simulink model "Gyro_Reading"  (R2022b)
settings: Solver=FixedStepDiscrete  StartTime=0.0  StopTime=inf  RelTol=1e-3  EnableMultiTasking=on
InitFcn:
  | run("InitScript.m");
undefined symbols (not defined in the file or in its folder): A_cal, b_cal, ODR, operatingFrequency
libraries: hdlsllib x12, mbedblockslib x10, simulink x6, aerolibanim x1
settings Model: ExtModeTrigDuration=10  Creator=rutrl  LastModifiedBy=rutrl
settings OptimizationCC: EnhancedBackFolding=on  PassReuseOutputArgsAs=Individual arguments  ZeroExternalMemoryAtStartup=off  ZeroInternalMemoryAtStartup=off  MaxStackSize=64  OptimizeBlockOrder=speed  DifferentSizesBufferReuse=on  OptimizationCustomize=off  EfficientTunableParamExpr=on
settings DebuggingCC: ParameterTunabilityLossMsg=error
settings HardwareCC: ProdBitPerPointer=32  ProdBitPerSizeT=32  ProdBitPerPtrDiffT=32  ProdLargestAtomicInteger=Long  ProdLargestAtomicFloat=Double  ProdWordSize=32  ProdLongLongMode=on  ProdHWDeviceType=ARM Compatible->ARM Cortex  UseEmbeddedCoderFeatures=off
settings SFSimCC: MATLABDynamicMemAlloc=off
settings RTWCC: Description=Embedded Coder  SystemTargetFile=ert.tlc  HardwareBoard=STM32 Nucleo L476RG  TLCOptions=-aInlineSetEventsForThisBaseRateFcn=TLC_FALSE -aSuppressMultiTaskScheduler=TLC_FALSE -aRateBasedStepFcn=1  TemplateMakefile=ert_default_tmf  Toolchain=GNU Tools for ARM Embedded Processors
settings CodeAppCC: ForceParamTrailComments=on  IgnoreCustomStorageClasses=off  OperatorAnnotations=on  SimulinkDataObjDesc=on  SFDataObjDesc=on  InsertBlockDesc=on
settings ERTTargetCC: SupportNonInlinedSFcns=on  ExtModeTransport=3  ExtModeStaticAlloc=on  ExtModeStaticAllocSize=2000  ExtModeMexFile=ext_xcp  ExtModeIntrfLevel=Level2 - Open

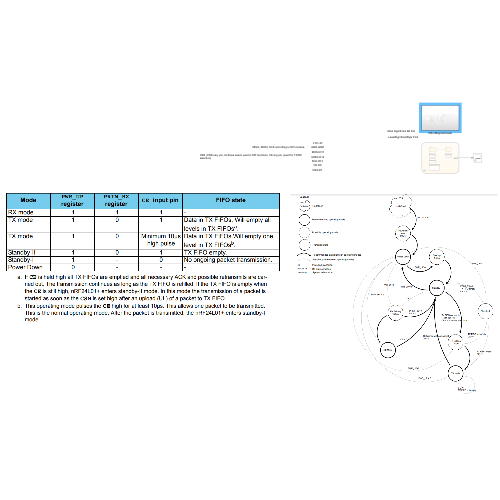
[thumbnail: Simulink's stored preview of the top-level diagram]
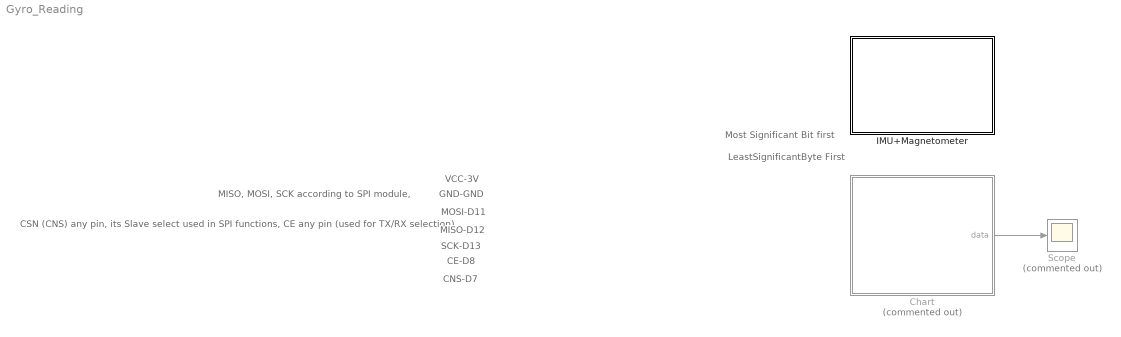
== system Gyro_Reading ==
  note: LeastSignificantByte First
  note: CNS-D7
  note: CSN (CNS) any pin, its Slave select used in SPI functions, CE any pin (used for TX/RX selection)
  note: MISO, MOSI, SCK according to SPI module,
  note: Most Significant Bit first
  note: CE-D8
  note: SCK-D13
  note: MISO-D12
  note: MOSI-D11
  note: GND-GND
  note: VCC-3V
  Chart : Stateflow chart  Commented=on  TreatAsAtomicUnit=on
  IMU+Magnetometer : Subsystem
  Scope : Scope  Commented=on
  wires:
  Chart/1(data) -> Scope/1

== system Gyro_Reading/Chart/? ==
  f : TriggerPort  TriggerType=function-call  VariantControl=(inherit)
      settings: CopyFcn=Stateflow.SLINSF.SimulinkMan.removeBlockPreDeleteFcn  PreDeleteFcn=Stateflow.SLINSF.SimulinkMan.unsafePredeleteFcn

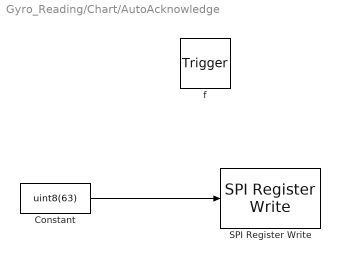
== system Gyro_Reading/Chart/AutoAcknowledge ==
  f : TriggerPort  TriggerType=function-call  VariantControl=(inherit)
      settings: CopyFcn=Stateflow.SLINSF.SimulinkMan.removeBlockPreDeleteFcn  PreDeleteFcn=Stateflow.SLINSF.SimulinkMan.unsafePredeleteFcn
  Constant : Constant  Value=uint8(63)
  SPI Register Write : mbedblockslib/SPI Register Write  SPIModule=0  Mode=Master  BusSpeed=uint32( 1000000 )  Pin=D7  FirstBitToTransfer=Most significant bit (MSB)  ClockMode=0  BlockFunction=Write  RegisterAddress=uint8(hex2dec('01'))  OutputDataType=int8  OutputDataLength=1  UseCustomSSPin=Explicit GPIO calls  ActiveLowSSPin=Active low
      settings: LibrarySourceBlock=stmnucleorootlib/Common/SPI Register Write
  wires:
  Constant/1 -> SPI Register Write/1

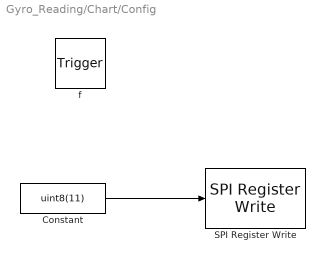
== system Gyro_Reading/Chart/Config ==
  f : TriggerPort  TriggerType=function-call  VariantControl=(inherit)
      settings: CopyFcn=Stateflow.SLINSF.SimulinkMan.removeBlockPreDeleteFcn  PreDeleteFcn=Stateflow.SLINSF.SimulinkMan.unsafePredeleteFcn
  Constant : Constant  Value=uint8(11)
  SPI Register Write : mbedblockslib/SPI Register Write  SPIModule=0  Mode=Master  BusSpeed=uint32( 1000000 )  Pin=D7  FirstBitToTransfer=Most significant bit (MSB)  ClockMode=0  BlockFunction=Write  RegisterAddress=uint8(hex2dec('00'))  OutputDataType=int8  OutputDataLength=1  UseCustomSSPin=Explicit GPIO calls  ActiveLowSSPin=Active low
      settings: LibrarySourceBlock=stmnucleorootlib/Common/SPI Register Write
  wires:
  Constant/1 -> SPI Register Write/1

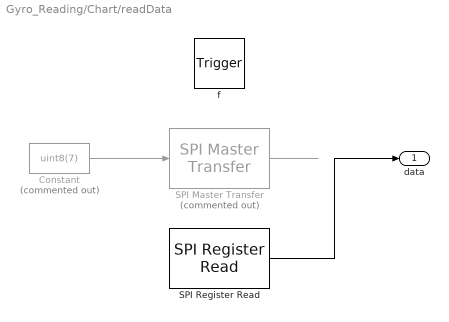
== system Gyro_Reading/Chart/readData ==
  f : TriggerPort  TriggerType=function-call  VariantControl=(inherit)
      settings: CopyFcn=Stateflow.SLINSF.SimulinkMan.removeBlockPreDeleteFcn  PreDeleteFcn=Stateflow.SLINSF.SimulinkMan.unsafePredeleteFcn
  Constant : Constant  Commented=on  Value=uint8(7)
  SPI Master Transfer : mbedblockslib/SPI Master Transfer  Commented=on  SPIModule=0  Mode=Master  BusSpeed=uint32( 1000000 )  Pin=D7  FirstBitToTransfer=Most significant bit (MSB)  ClockMode=0  BlockFunction=Transfer  RegisterAddress=0  OutputDataType=int8  OutputDataLength=1  UseCustomSSPin=Explicit GPIO calls  ActiveLowSSPin=Active low
      settings: LibrarySourceBlock=stmnucleorootlib/Common/SPI Master Transfer
  SPI Register Read : mbedblockslib/SPI Register Read  SPIModule=0  Mode=Master  BusSpeed=uint32( 1000000 )  Pin=D7  FirstBitToTransfer=Most significant bit (MSB)  ClockMode=0  BlockFunction=Read  RegisterAddress=uint8(hex2dec('07'))  OutputDataType=uint8  OutputDataLength=1  SampleTime=-1  UseCustomSSPin=Explicit GPIO calls  ActiveLowSSPin=Active low
      settings: LibrarySourceBlock=stmnucleorootlib/Common/SPI Register Read
  data : Outport
  wires:
  SPI Master Transfer/1 -> ?
  Constant/1 -> SPI Master Transfer/1
  SPI Register Read/1 -> data/1

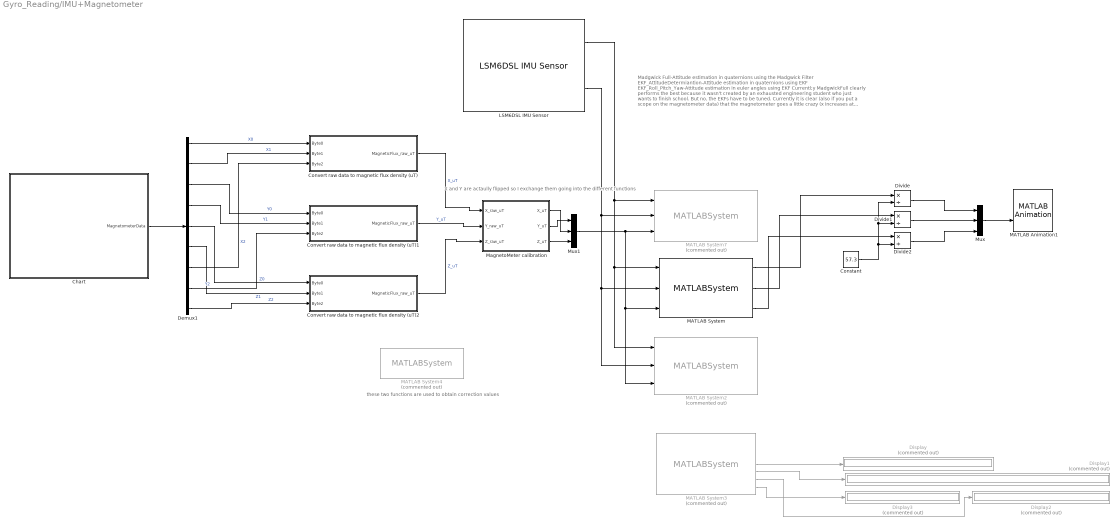
== system Gyro_Reading/IMU+Magnetometer ==
  note: Madgwick Full-Attitude estimation in quaternions using the Madgwick Filter
      | EKF_AttitudeDetermiantion-Attitude estimation in quaternions using EKF
      | EKF_Roll_Pitch_Yaw-Attitude estimation in euler angles using EKF
      |
      | Currentl;y MadgwickFull clearly performs the best because it wasn't created by
      | an exhausted engineering student who just wants to finish school. But no, the
      | EKFs have to be tuned. Currently it is clear (also if you put a scope on the
      | magnetometer data) that the magnetometer goes a little crazy (x increases at higher rate than y (or the other way around) so it mathematically results in change of yaw but then it settles at the appropriate values again once the speed decreases) at higher angular speeds.
      | Hence it is worth the time to try to come up with a function that will estiamte the most appropriate Q and R values based on the angular speed, such that at higher speeds we rely more on the gyroscope (prediction) and at lower speed we rely more on the magnetometer (update)
      |
      | In conclusion, these can be used as prrof of concept for further development.
  note: X and Y are actaully flipped so I exchange them going into the different functions
  note: these two functions are used to obtain correction values
  Chart : Stateflow chart  TreatAsAtomicUnit=on
  Constant : Constant  Value=57.3
  Convert raw data to magnetic flux density (uT) : Subsystem
  Convert raw data to magnetic flux density (uT)1 : Subsystem
  Convert raw data to magnetic flux density (uT)2 : Subsystem
  Demux1 : Demux  Outputs=9
  Display{,1..3} (4 alike) : Display  Commented=on
  Divide : Product  Inputs=*/
  Divide1 : Product  Inputs=*/
  Divide2 : Product  Inputs=*/
  LSM6DSL IMU Sensor : mbedblockslib/LSM6DSL IMU Sensor  I2CModule=0  I2CAddress=0x6A  IsActiveAcceleration=on  IsActiveAngularRate=on  IsActiveTemperature=off  IsActiveStatus=off  IsActiveTimeStamp=off  SampleTime=1/operatingFrequency  QueueSizeFactor=3  AccelerometerRange=+/- 8g  AccelerometerODR=208 Hz  AccelLPF1BW=ODR/4  AccelSelectCompositeFilter=Low pass filter  AccelLPF2BW=ODR/100  AccelHPFBW=ODR/100  GyroscopeRange=1000 dps  GyroscopeODR=208 Hz  EnableGyroHPF=off  GyroHPFBW=0.016 Hz  EnableGyroLPF=on  GyroLPFBWMode=3
      settings: LibrarySourceBlock=stmnucleosensorslib/LSM6DSL IMU Sensor
  MATLAB Animation1 : aerolibanim/MATLAB Animation  Tag=Matlab Animation 6 DOF  Vehicles=1  Geometries='astredwedge.mat'  BoundingBoxCoordinates=[-50,50,-50,50,-50,50]  CameraOffset=[-150,-50,0]  CameraViewAngle=3  SampleTime=-1  FigurePosition=[529,285,1158,525]
  MATLAB System : MATLABSystem  System=EKF_AttitudeDetermination  samplingFrequency=operatingFrequency  gyro_x_corr=gyro_x_corr  gyro_y_corr=gyro_y_corr  gyro_z_corr=gyro_z_corr  SimulateUsing=Code generation
      mask Type: EKF_AttitudeDetermination
      mask Display:
      | disp('EKF_AttitudeDetermination');
      | port_label('input',1,'accelerometer');
      | port_label('input',2,'gyroscope');
      | port_label('input',3,'magnetometer');
      | port_label('output',1,'roll');
      | port_label('output',2,'pitch');
      | port_label('output',3,'yaw');
  MATLAB System2 : MATLABSystem  Commented=on  System=EKF_Roll_Pitch_Yaw  samplingFrequency=operatingFrequency  gyro_x_corr=gyro_x_corr  gyro_y_corr=gyro_y_corr  gyro_z_corr=gyro_z_corr  SimulateUsing=Code generation
      mask Type: EKF_Roll_Pitch_Yaw
      mask Display:
      | disp('EKF_Roll_Pitch_Yaw');
      | port_label('input',1,'accelerometer');
      | port_label('input',2,'gyroscope');
      | port_label('input',3,'magnetometer');
      | port_label('output',1,'roll');
      | port_label('output',2,'pitch');
      | port_label('output',3,'yaw');
  MATLAB System3 : MATLABSystem  Commented=on  System=EKF_Testing  samplingFrequency=operatingFrequency  gyro_x_corr=gyro_x_corr  gyro_y_corr=gyro_y_corr  gyro_z_corr=gyro_z_corr  SimulateUsing=Code generation
      mask Type: EKF_Testing
      mask Display:
      | disp('EKF_Testing');
      | port_label('input',1,'accelerometer');
      | port_label('input',2,'gyroscope');
      | port_label('input',3,'magnetometer');
      | port_label('output',1,'roll');
      | port_label('output',2,'pitch');
      | port_label('output',3,'yaw');
      | port_label('output',4,'q');
      | port_label('output',5,'h');
      | port_label('output',6,'m_prime');
      | port_label('output',7,'a');
  MATLAB System4 : MATLABSystem  Commented=on  System=GyroCorr  operatingFrequency=operatingFrequency  SimulateUsing=Code generation
      mask Type: GyroCorr
      mask Display:
      | disp('GyroCorr');
      | port_label('input',1,'gyroscope');
      | port_label('output',1,'gyro_x');
      | port_label('output',2,'gyro_y');
      | port_label('output',3,'gyro_z');
  MATLAB System7 : MATLABSystem  Commented=on  System=MadgwickFull  samplingFrequency=operatingFrequency  gyro_x_corr=gyro_x_corr  gyro_y_corr=gyro_y_corr  gyro_z_corr=gyro_z_corr  SimulateUsing=Code generation
      mask Type: MadgwickFull
      mask Display:
      | disp('MadgwickFull');
      | port_label('input',1,'accelerometer');
      | port_label('input',2,'gyroscope');
      | port_label('input',3,'magnetometer');
      | port_label('output',1,'roll');
      | port_label('output',2,'pitch');
      | port_label('output',3,'yaw');
  MagnetoMeter calibration : Subsystem
  Mux : Mux  Inputs=3
  Mux1 : Mux  Inputs=3
  wires:
  Demux1/5 -> Convert raw data to magnetic flux density (uT)2/1(Byte0)  "Z0"
  Demux1/9 -> Convert raw data to magnetic flux density (uT)2/3(Byte2)  "Z2"
  Convert raw data to magnetic flux density (uT)2/1(MagneticFlux_raw_uT) -> MagnetoMeter calibration/3(Z_raw_uT)  "Z_uT"
  Demux1/4 -> Convert raw data to magnetic flux density (uT)1/2(Byte1)  "Y1"
  Convert raw data to magnetic flux density (uT)/1(MagneticFlux_raw_uT) -> MagnetoMeter calibration/1(X_raw_uT)  "X_uT"
  Demux1/6 -> Convert raw data to magnetic flux density (uT)2/2(Byte1)  "Z1"
  Demux1/1 -> Convert raw data to magnetic flux density (uT)/1(Byte0)  "X0"
  Demux1/7 -> Convert raw data to magnetic flux density (uT)/3(Byte2)  "X2"
  Convert raw data to magnetic flux density (uT)1/1(MagneticFlux_raw_uT) -> MagnetoMeter calibration/2(Y_raw_uT)  "Y_uT"
  Demux1/8 -> Convert raw data to magnetic flux density (uT)1/3(Byte2)  "Y2"
  Demux1/2 -> Convert raw data to magnetic flux density (uT)/2(Byte1)  "X1"
  Chart/1(MagnetometerData) -> Demux1/1
  Demux1/3 -> Convert raw data to magnetic flux density (uT)1/1(Byte0)  "Y0"
  LSM6DSL IMU Sensor/2 -> MATLAB System7/2, MATLAB System/2, MATLAB System2/2
  LSM6DSL IMU Sensor/1 -> MATLAB System7/1, MATLAB System/1, MATLAB System2/1
  Constant/1 -> Divide/2, Divide1/2, Divide2/2
  Divide1/1 -> Mux/2
  MagnetoMeter calibration/1(X_uT) -> Mux1/2
  MagnetoMeter calibration/2(Y_uT) -> Mux1/1
  MagnetoMeter calibration/3(Z_uT) -> Mux1/3
  Mux/1 -> MATLAB Animation1/2
  Divide/1 -> Mux/1
  Divide2/1 -> Mux/3
  MATLAB System3/4 -> Display/1
  MATLAB System3/5 -> Display1/1
  MATLAB System3/6 -> Display2/1
  MATLAB System3/7 -> Display3/1
  Mux1/1 -> MATLAB System2/3, MATLAB System/3, MATLAB System7/3
  MATLAB System/1 -> Divide/1
  MATLAB System/2 -> Divide1/1
  MATLAB System/3 -> Divide2/1

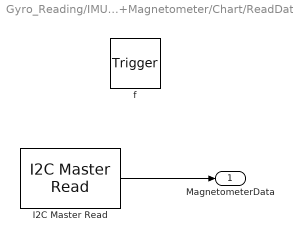
== system Gyro_Reading/IMU+Magnetometer/Chart/ReadData ==
  f : TriggerPort  TriggerType=function-call  VariantControl=(inherit)
      settings: CopyFcn=Stateflow.SLINSF.SimulinkMan.removeBlockPreDeleteFcn  PreDeleteFcn=Stateflow.SLINSF.SimulinkMan.unsafePredeleteFcn
  I2C Master Read : mbedblockslib/I2C Master Read  I2CModule=0  Mode=Master  SlaveAddress=hex2dec('30')  SlaveByteOrder=LittleEndian  Direction=Receiver  RegisterAddressMode=on  RegisterAddress=uint8(hex2dec('00'))  SlaveDataType=uint8  DataLength=9  NoAck=off  RepeatedStart=off  OutputStatus=off  SampleTime=-1
      settings: LibrarySourceBlock=stmnucleorootlib/Common/I2C Master Read
  MagnetometerData : Outport
  wires:
  I2C Master Read/1 -> MagnetometerData/1

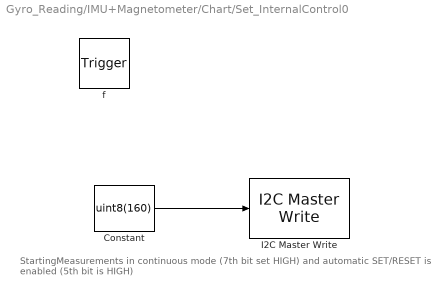
== system Gyro_Reading/IMU+Magnetometer/Chart/Set_InternalControl0 ==
  note: StartingMeasurements in continuous mode (7th bit set HIGH) and automatic SET/RESET is enabled (5th bit is HIGH)
  f : TriggerPort  TriggerType=function-call  VariantControl=(inherit)
      settings: CopyFcn=Stateflow.SLINSF.SimulinkMan.removeBlockPreDeleteFcn  PreDeleteFcn=Stateflow.SLINSF.SimulinkMan.unsafePredeleteFcn
  Constant : Constant  Value=uint8(160)
  I2C Master Write : mbedblockslib/I2C Master Write  I2CModule=0  Mode=Master  SlaveAddress=hex2dec('30')  SlaveByteOrder=BigEndian  Direction=Transmitter  RegisterAddressMode=on  RegisterAddress=uint8(hex2dec('1B'))  SlaveDataType=uint8  DataLength=2  NoAck=off  RepeatedStart=off  OutputStatus=off
      settings: LibrarySourceBlock=stmnucleorootlib/Common/I2C Master Write
  wires:
  Constant/1 -> I2C Master Write/1

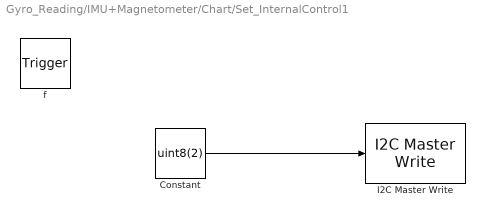
== system Gyro_Reading/IMU+Magnetometer/Chart/Set_InternalControl1 ==
  f : TriggerPort  TriggerType=function-call  VariantControl=(inherit)
      settings: CopyFcn=Stateflow.SLINSF.SimulinkMan.removeBlockPreDeleteFcn  PreDeleteFcn=Stateflow.SLINSF.SimulinkMan.unsafePredeleteFcn
  Constant : Constant  Value=uint8(2)
  I2C Master Write : mbedblockslib/I2C Master Write  I2CModule=0  Mode=Master  SlaveAddress=hex2dec('30')  SlaveByteOrder=BigEndian  Direction=Transmitter  RegisterAddressMode=on  RegisterAddress=uint8(hex2dec('1C'))  SlaveDataType=uint8  DataLength=2  NoAck=off  RepeatedStart=off  OutputStatus=off
      settings: LibrarySourceBlock=stmnucleorootlib/Common/I2C Master Write
  wires:
  Constant/1 -> I2C Master Write/1

== system Gyro_Reading/IMU+Magnetometer/Chart/Set_InternalControl2 ==
  note: Just setting continuous mode to 1
  f : TriggerPort  TriggerType=function-call  VariantControl=(inherit)
      settings: CopyFcn=Stateflow.SLINSF.SimulinkMan.removeBlockPreDeleteFcn  PreDeleteFcn=Stateflow.SLINSF.SimulinkMan.unsafePredeleteFcn
  Constant : Constant  Value=uint8(16)
  I2C Master Write : mbedblockslib/I2C Master Write  I2CModule=0  Mode=Master  SlaveAddress=hex2dec('30')  SlaveByteOrder=BigEndian  Direction=Transmitter  RegisterAddressMode=on  RegisterAddress=uint8(hex2dec('1D'))  SlaveDataType=uint8  DataLength=2  NoAck=off  RepeatedStart=off  OutputStatus=off
      settings: LibrarySourceBlock=stmnucleorootlib/Common/I2C Master Write
  wires:
  Constant/1 -> I2C Master Write/1

== system Gyro_Reading/IMU+Magnetometer/Chart/Set_ODR ==
  note: Just put desired frequency into bracket. BW is set to 10 in internal control 1
  f : TriggerPort  TriggerType=function-call  VariantControl=(inherit)
      settings: CopyFcn=Stateflow.SLINSF.SimulinkMan.removeBlockPreDeleteFcn  PreDeleteFcn=Stateflow.SLINSF.SimulinkMan.unsafePredeleteFcn
  Constant : Constant  Value=uint8(200)
  I2C Master Write : mbedblockslib/I2C Master Write  I2CModule=0  Mode=Master  SlaveAddress=hex2dec('30')  SlaveByteOrder=BigEndian  Direction=Transmitter  RegisterAddressMode=on  RegisterAddress=uint8(hex2dec('1A'))  SlaveDataType=uint8  DataLength=2  NoAck=off  RepeatedStart=off  OutputStatus=off
      settings: LibrarySourceBlock=stmnucleorootlib/Common/I2C Master Write
  wires:
  Constant/1 -> I2C Master Write/1

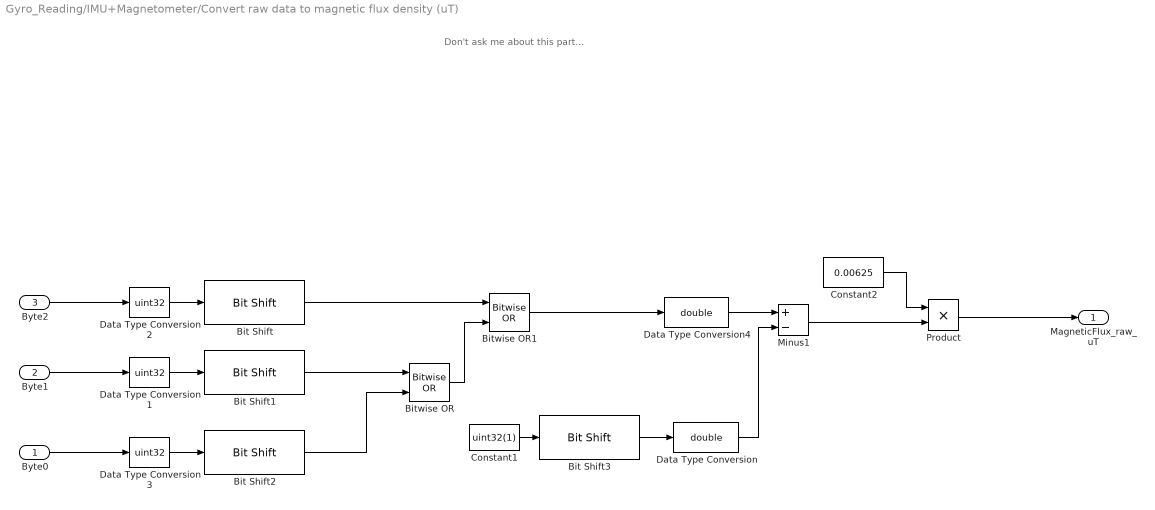
== system Gyro_Reading/IMU+Magnetometer/Convert raw data to magnetic flux density (uT) ==
  note: Don't ask me about this part...
  Byte0 : Inport
  Byte1 : Inport  Port=2
  Byte2 : Inport  Port=3
  Bit Shift : hdlsllib/Logic and Bit Operations/Bit Shift  mode=Shift Right Logical  N=4
  Bit Shift1 : hdlsllib/Logic and Bit Operations/Bit Shift  mode=Shift Left Logical  N=4
  Bit Shift2 : hdlsllib/Logic and Bit Operations/Bit Shift  mode=Shift Left Logical  N=12
  Bit Shift3 : hdlsllib/Logic and Bit Operations/Bit Shift  mode=Shift Left Logical  N=19
  Bitwise OR : simulink/Logic and Bit Operations/Bitwise Operator  logicop=OR  UseBitMask=off  NumInputPorts=2  BitMask=bin2dec('11011001')  BitMaskRealWorld=Stored Integer
      settings: LibrarySourceBlock=|
      | simulink/Quick Insert/Logic and Bit
      | Operations/Bitwise OR
  Bitwise OR1 : simulink/Logic and Bit Operations/Bitwise Operator  logicop=OR  UseBitMask=off  NumInputPorts=2  BitMask=bin2dec('11011001')  BitMaskRealWorld=Stored Integer
      settings: LibrarySourceBlock=|
      | simulink/Quick Insert/Logic and Bit
      | Operations/Bitwise OR
  Constant1 : Constant  Value=uint32(1)
  Constant2 : Constant  Value=0.00625
  Data Type Conversion : DataTypeConversion  OutDataTypeStr=double  SaturateOnIntegerOverflow=off  RndMeth=Floor
  Data Type Conversion1 : DataTypeConversion  OutDataTypeStr=uint32  SaturateOnIntegerOverflow=off  RndMeth=Floor
  Data Type Conversion2 : DataTypeConversion  OutDataTypeStr=uint32  SaturateOnIntegerOverflow=off  RndMeth=Floor
  Data Type Conversion3 : DataTypeConversion  OutDataTypeStr=uint32  SaturateOnIntegerOverflow=off  RndMeth=Floor
  Data Type Conversion4 : DataTypeConversion  OutDataTypeStr=double  SaturateOnIntegerOverflow=off  RndMeth=Floor
  Minus1 : Sum  Inputs=+-
  Product : Product
  MagneticFlux_raw_uT : Outport
  wires:
  Bit Shift/1 -> Bitwise OR1/1
  Bit Shift2/1 -> Bitwise OR/2
  Data Type Conversion3/1 -> Bit Shift2/1
  Byte0/1 -> Data Type Conversion3/1
  Bit Shift1/1 -> Bitwise OR/1
  Bitwise OR1/1 -> Data Type Conversion4/1
  Constant1/1 -> Bit Shift3/1
  Bitwise OR/1 -> Bitwise OR1/2
  Data Type Conversion2/1 -> Bit Shift/1
  Minus1/1 -> Product/2
  Byte1/1 -> Data Type Conversion1/1
  Bit Shift3/1 -> Data Type Conversion/1
  Data Type Conversion1/1 -> Bit Shift1/1
  Product/1 -> MagneticFlux_raw_uT/1
  Constant2/1 -> Product/1
  Byte2/1 -> Data Type Conversion2/1
  Data Type Conversion/1 -> Minus1/2
  Data Type Conversion4/1 -> Minus1/1

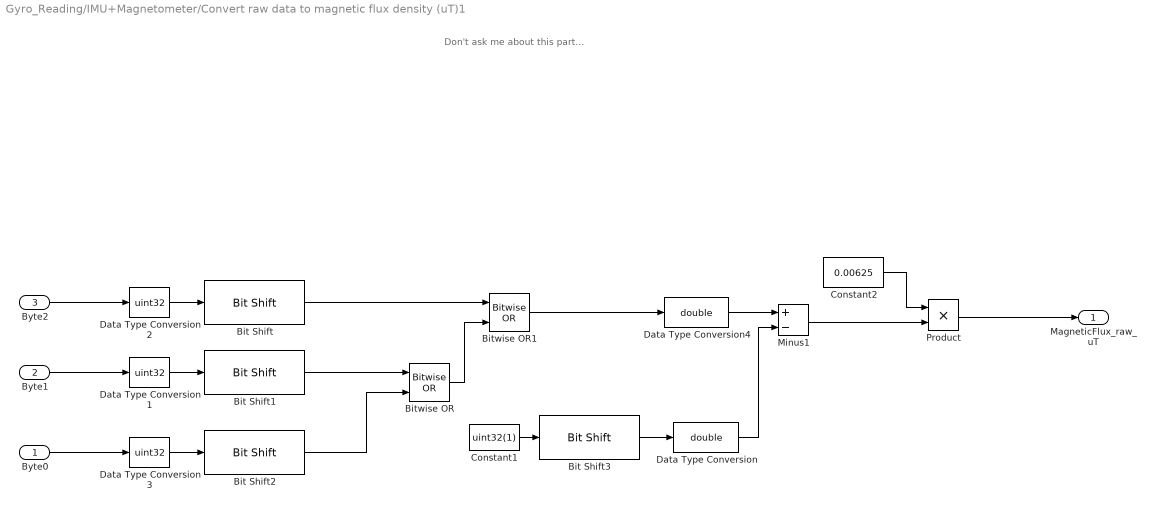
== system Gyro_Reading/IMU+Magnetometer/Convert raw data to magnetic flux density (uT)1 ==
  note: Don't ask me about this part...
  Byte0 : Inport
  Byte1 : Inport  Port=2
  Byte2 : Inport  Port=3
  Bit Shift : hdlsllib/Logic and Bit Operations/Bit Shift  mode=Shift Right Logical  N=4
  Bit Shift1 : hdlsllib/Logic and Bit Operations/Bit Shift  mode=Shift Left Logical  N=4
  Bit Shift2 : hdlsllib/Logic and Bit Operations/Bit Shift  mode=Shift Left Logical  N=12
  Bit Shift3 : hdlsllib/Logic and Bit Operations/Bit Shift  mode=Shift Left Logical  N=19
  Bitwise OR : simulink/Logic and Bit Operations/Bitwise Operator  logicop=OR  UseBitMask=off  NumInputPorts=2  BitMask=bin2dec('11011001')  BitMaskRealWorld=Stored Integer
      settings: LibrarySourceBlock=|
      | simulink/Quick Insert/Logic and Bit
      | Operations/Bitwise OR
  Bitwise OR1 : simulink/Logic and Bit Operations/Bitwise Operator  logicop=OR  UseBitMask=off  NumInputPorts=2  BitMask=bin2dec('11011001')  BitMaskRealWorld=Stored Integer
      settings: LibrarySourceBlock=|
      | simulink/Quick Insert/Logic and Bit
      | Operations/Bitwise OR
  Constant1 : Constant  Value=uint32(1)
  Constant2 : Constant  Value=0.00625
  Data Type Conversion : DataTypeConversion  OutDataTypeStr=double  SaturateOnIntegerOverflow=off  RndMeth=Floor
  Data Type Conversion1 : DataTypeConversion  OutDataTypeStr=uint32  SaturateOnIntegerOverflow=off  RndMeth=Floor
  Data Type Conversion2 : DataTypeConversion  OutDataTypeStr=uint32  SaturateOnIntegerOverflow=off  RndMeth=Floor
  Data Type Conversion3 : DataTypeConversion  OutDataTypeStr=uint32  SaturateOnIntegerOverflow=off  RndMeth=Floor
  Data Type Conversion4 : DataTypeConversion  OutDataTypeStr=double  SaturateOnIntegerOverflow=off  RndMeth=Floor
  Minus1 : Sum  Inputs=+-
  Product : Product
  MagneticFlux_raw_uT : Outport
  wires:
  Bit Shift/1 -> Bitwise OR1/1
  Bit Shift2/1 -> Bitwise OR/2
  Data Type Conversion3/1 -> Bit Shift2/1
  Byte0/1 -> Data Type Conversion3/1
  Bit Shift1/1 -> Bitwise OR/1
  Bitwise OR1/1 -> Data Type Conversion4/1
  Constant1/1 -> Bit Shift3/1
  Bitwise OR/1 -> Bitwise OR1/2
  Data Type Conversion2/1 -> Bit Shift/1
  Minus1/1 -> Product/2
  Byte1/1 -> Data Type Conversion1/1
  Bit Shift3/1 -> Data Type Conversion/1
  Data Type Conversion1/1 -> Bit Shift1/1
  Product/1 -> MagneticFlux_raw_uT/1
  Constant2/1 -> Product/1
  Byte2/1 -> Data Type Conversion2/1
  Data Type Conversion/1 -> Minus1/2
  Data Type Conversion4/1 -> Minus1/1

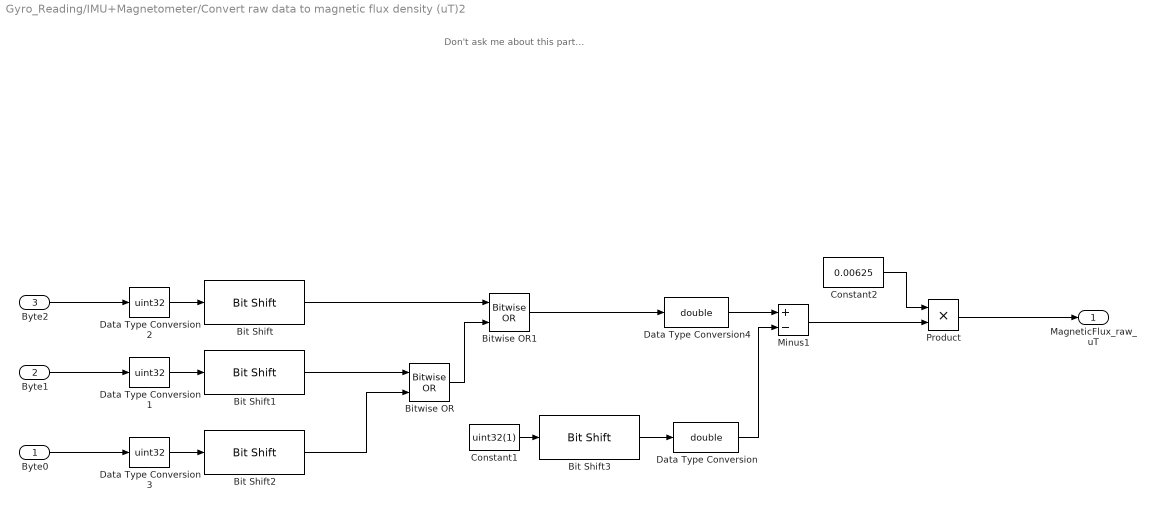
== system Gyro_Reading/IMU+Magnetometer/Convert raw data to magnetic flux density (uT)2 ==
  note: Don't ask me about this part...
  Byte0 : Inport
  Byte1 : Inport  Port=2
  Byte2 : Inport  Port=3
  Bit Shift : hdlsllib/Logic and Bit Operations/Bit Shift  mode=Shift Right Logical  N=4
  Bit Shift1 : hdlsllib/Logic and Bit Operations/Bit Shift  mode=Shift Left Logical  N=4
  Bit Shift2 : hdlsllib/Logic and Bit Operations/Bit Shift  mode=Shift Left Logical  N=12
  Bit Shift3 : hdlsllib/Logic and Bit Operations/Bit Shift  mode=Shift Left Logical  N=19
  Bitwise OR : simulink/Logic and Bit Operations/Bitwise Operator  logicop=OR  UseBitMask=off  NumInputPorts=2  BitMask=bin2dec('11011001')  BitMaskRealWorld=Stored Integer
      settings: LibrarySourceBlock=|
      | simulink/Quick Insert/Logic and Bit
      | Operations/Bitwise OR
  Bitwise OR1 : simulink/Logic and Bit Operations/Bitwise Operator  logicop=OR  UseBitMask=off  NumInputPorts=2  BitMask=bin2dec('11011001')  BitMaskRealWorld=Stored Integer
      settings: LibrarySourceBlock=|
      | simulink/Quick Insert/Logic and Bit
      | Operations/Bitwise OR
  Constant1 : Constant  Value=uint32(1)
  Constant2 : Constant  Value=0.00625
  Data Type Conversion : DataTypeConversion  OutDataTypeStr=double  SaturateOnIntegerOverflow=off  RndMeth=Floor
  Data Type Conversion1 : DataTypeConversion  OutDataTypeStr=uint32  SaturateOnIntegerOverflow=off  RndMeth=Floor
  Data Type Conversion2 : DataTypeConversion  OutDataTypeStr=uint32  SaturateOnIntegerOverflow=off  RndMeth=Floor
  Data Type Conversion3 : DataTypeConversion  OutDataTypeStr=uint32  SaturateOnIntegerOverflow=off  RndMeth=Floor
  Data Type Conversion4 : DataTypeConversion  OutDataTypeStr=double  SaturateOnIntegerOverflow=off  RndMeth=Floor
  Minus1 : Sum  Inputs=+-
  Product : Product
  MagneticFlux_raw_uT : Outport
  wires:
  Bit Shift/1 -> Bitwise OR1/1
  Bit Shift2/1 -> Bitwise OR/2
  Data Type Conversion3/1 -> Bit Shift2/1
  Byte0/1 -> Data Type Conversion3/1
  Bit Shift1/1 -> Bitwise OR/1
  Bitwise OR1/1 -> Data Type Conversion4/1
  Constant1/1 -> Bit Shift3/1
  Bitwise OR/1 -> Bitwise OR1/2
  Data Type Conversion2/1 -> Bit Shift/1
  Minus1/1 -> Product/2
  Byte1/1 -> Data Type Conversion1/1
  Bit Shift3/1 -> Data Type Conversion/1
  Data Type Conversion1/1 -> Bit Shift1/1
  Product/1 -> MagneticFlux_raw_uT/1
  Constant2/1 -> Product/1
  Byte2/1 -> Data Type Conversion2/1
  Data Type Conversion/1 -> Minus1/2
  Data Type Conversion4/1 -> Minus1/1

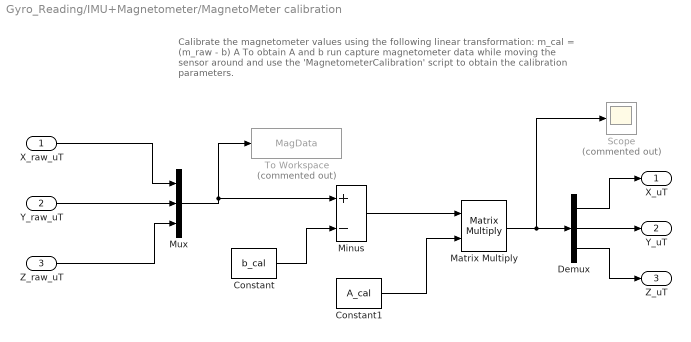
== system Gyro_Reading/IMU+Magnetometer/MagnetoMeter calibration ==
  note: Calibrate the magnetometer values using the following linear transformation:
      | m_cal = (m_raw - b) A
      |
      | To obtain A and b run capture magnetometer data while moving the sensor around
      | and use the 'MagnetometerCalibration' script to obtain the calibration parameters.
  X_raw_uT : Inport
  Y_raw_uT : Inport  Port=2
  Z_raw_uT : Inport  Port=3
  Constant : Constant  Value=b_cal
  Constant1 : Constant  Value=A_cal
  Demux : Demux  Outputs=3
  Matrix Multiply : Product  Multiplication=Matrix(*)
  Minus : Sum  Inputs=+-
  Mux : Mux  Inputs=3
  Scope : Scope  Commented=on
  To Workspace : ToWorkspace  Commented=on  VariableName=MagData  SaveFormat=Timeseries  SampleTime=-1
  X_uT : Outport
  Y_uT : Outport  Port=2
  Z_uT : Outport  Port=3
  wires:
  Minus/1 -> Matrix Multiply/1
  Mux/1 -> To Workspace/1, Minus/1
  Z_raw_uT/1 -> Mux/3
  Constant/1 -> Minus/2
  Y_raw_uT/1 -> Mux/2
  X_raw_uT/1 -> Mux/1
  Constant1/1 -> Matrix Multiply/2
  Matrix Multiply/1 -> Scope/1, Demux/1
  Demux/3 -> Z_uT/1
  Demux/1 -> X_uT/1
  Demux/2 -> Y_uT/1

== stateflow chart Gyro_Reading/Chart ==
  state Set_up_
    Config();
    AutoAcknowledge();
  state Read_
    data = readData()
  state Config [function]
  state data = readData [function]
  state AutoAcknowledge [function]
  state ? [function]
  (default) -> Set_up_
  Set_up_ -> Read_ : [after(1,tick)]
  data: data function_output; data output

== stateflow chart Gyro_Reading/IMU+Magnetometer/Chart ==
  settings: updateMethod=DISCRETE  sampleTime=1/operatingFrequency
  note: The magnetometer uses Big Endian, so the most significant bit is sent first. So all communications needs to be set to BigEndian
  state Magnetometr_Setup_
    Set_InternalControl1();
    Set_ODR();
    Set_InternalControl0();
    Set_InternalControl2();
  state Read_Data_
    MagnetometerData=ReadData();
  state Set_InternalControl1 [function]
  state MagnetometerData = ReadData [function]
  state Set_ODR [function]
  state Set_InternalControl0 [function]
  state Set_InternalControl2 [function]
  (default) -> Magnetometr_Setup_
  Magnetometr_Setup_ -> Read_Data_ : [after(10,tick)]
  data: MagnetometerData function_output; MagnetometerData output
